simulink library "VUT_lib"  (R2023b)
settings: Solver=VariableStepAuto  StartTime=0.0  StopTime=10.0  RelTol=1e-3
undefined symbols (not defined in the file): zeroProtn
libraries: $bdroot x15
settings Model: Creator=blatak  LastModifiedBy=blatak
settings ModelReferenceCC: EnableRefExpFcnMdlSchedulingChecks=on

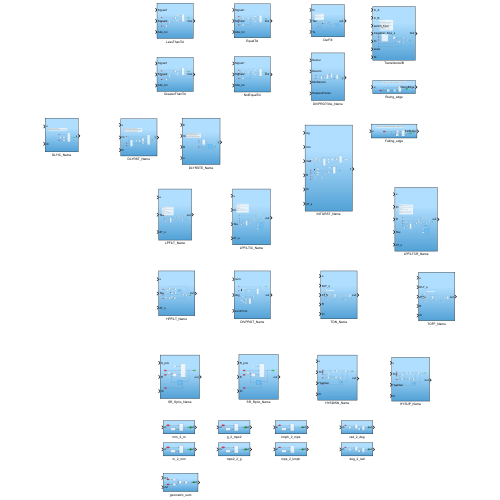
[thumbnail: Simulink's stored preview of the top-level diagram]
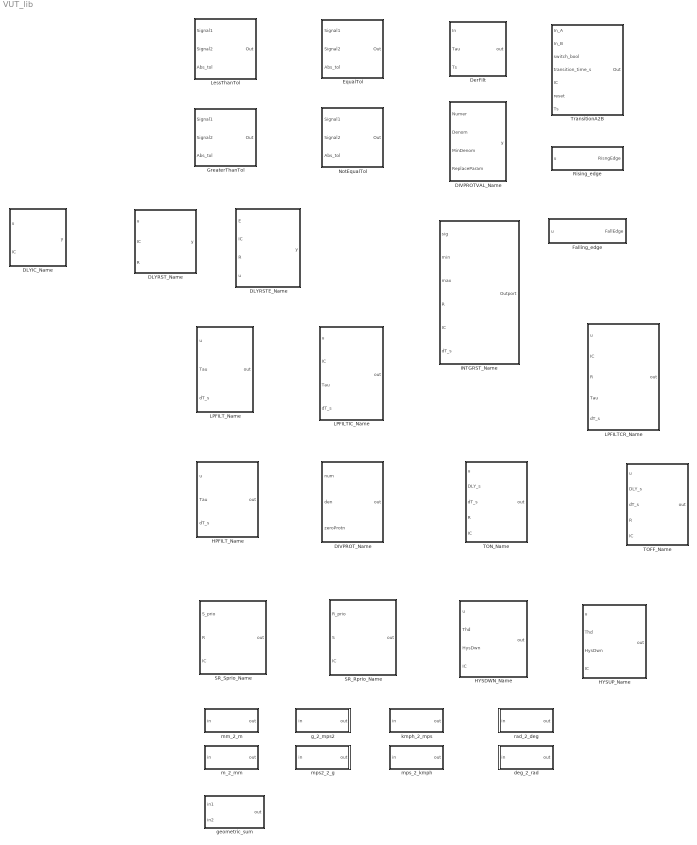
== system VUT_lib ==
  DIVPROTVAL_Name : Subsystem
  DIVPROT_Name : Subsystem
  DLYIC_Name : Subsystem
  DLYRSTE_Name : Subsystem
  DLYRST_Name : Subsystem
  DerFilt : Subsystem
  EqualTol : Subsystem
  Falling_edge : Subsystem
  GreaterThanTol : Subsystem
  HPFILT_Name : Subsystem
  HYSDWN_Name : Subsystem
  HYSUP_Name : Subsystem
  INTGRST_Name : Subsystem
  LPFILTCR_Name : Subsystem
  LPFILTIC_Name : Subsystem
  LPFILT_Name : Subsystem
  LessThanTol : Subsystem
  NotEqualTol : Subsystem
  Rising_edge : Subsystem
  SR_Rprio_Name : Subsystem
  SR_Sprio_Name : Subsystem
  TOFF_Name : Subsystem
  TON_Name : Subsystem
  TransitionA2B : Subsystem
  deg_2_rad : Subsystem
  g_2_mps2 : Subsystem
  geometric_sum : Subsystem
  kmph_2_mps : Subsystem
  m_2_mm : Subsystem
  mm_2_m : Subsystem
  mps2_2_g : Subsystem
  mps_2_kmph : Subsystem
  rad_2_deg : Subsystem

== system VUT_lib/DIVPROTVAL_Name ==
  Numer : Inport
  Denom : Inport  Port=2
  MinDenom : Inport  Port=3
  ReplaceParam : Inport  Port=4
  Abs : Abs  SaturateOnIntegerOverflow=off
  Constant : Constant  OutDataTypeStr=single
  Divide : Product  Inputs=*/  RndMeth=Zero  SaturateOnIntegerOverflow=on
  GreaterThan : RelationalOperator  Operator=>  OutDataTypeStr=boolean  RndMeth=Simplest  InputSameDT=off
  Switch : Switch  Criteria=u2 ~= 0  SaturateOnIntegerOverflow=off  InputSameDT=off
  Switch1 : Switch  Criteria=u2 ~= 0  SaturateOnIntegerOverflow=off  InputSameDT=off
  y : Outport
  wires:
  Abs/1 -> GreaterThan/1
  MinDenom/1 -> GreaterThan/2
  Constant/1 -> Switch/3
  Denom/1 -> Abs/1, Switch/1
  GreaterThan/1 -> Switch/2, Switch1/2
  Switch/1 -> Divide/2
  Numer/1 -> Divide/1
  Divide/1 -> Switch1/1
  Switch1/1 -> y/1
  ReplaceParam/1 -> Switch1/3

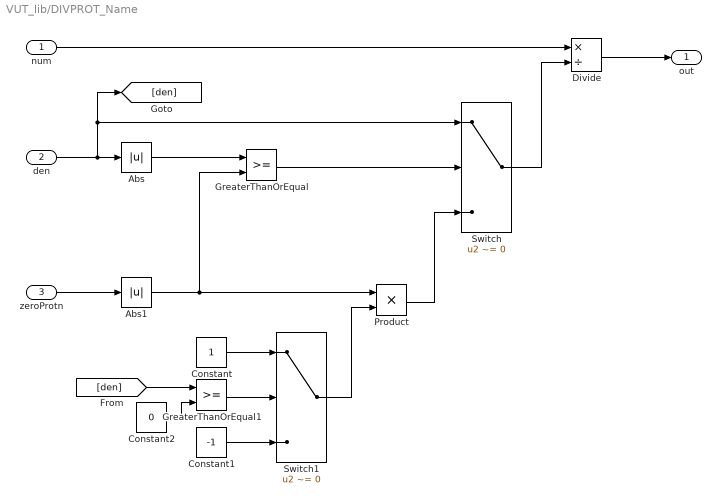
== system VUT_lib/DIVPROT_Name ==
  num : Inport
  den : Inport  Port=2
  zeroProtn : Inport  Port=3
  Abs : Abs  SaturateOnIntegerOverflow=off
  Abs1 : Abs  SaturateOnIntegerOverflow=off
  Constant : Constant  OutDataTypeStr=single
  Constant1 : Constant  Value=-1  OutDataTypeStr=single
  Constant2 : Constant  Value=0  OutDataTypeStr=single
  Divide : Product  Inputs=*/  RndMeth=Zero  SaturateOnIntegerOverflow=on
  GreaterThanOrEqual : RelationalOperator  OutDataTypeStr=boolean  RndMeth=Simplest  InputSameDT=off
  GreaterThanOrEqual1 : RelationalOperator  OutDataTypeStr=boolean  RndMeth=Simplest  InputSameDT=off
  Product : Product
  Switch : Switch  Criteria=u2 ~= 0  SaturateOnIntegerOverflow=off  InputSameDT=off
  Switch1 : Switch  Criteria=u2 ~= 0  SaturateOnIntegerOverflow=off  InputSameDT=off
  out : Outport
  wires:
  den/1 -> Switch/1, [den], Abs/1
  Abs/1 -> GreaterThanOrEqual/1
  zeroProtn/1 -> Abs1/1
  Abs1/1 -> Product/1, GreaterThanOrEqual/2
  GreaterThanOrEqual/1 -> Switch/2
  num/1 -> Divide/1
  Switch/1 -> Divide/2
  Divide/1 -> out/1
  Constant/1 -> Switch1/1
  Constant1/1 -> Switch1/3
  GreaterThanOrEqual1/1 -> Switch1/2
  [den] -> GreaterThanOrEqual1/1
  Constant2/1 -> GreaterThanOrEqual1/2
  Switch1/1 -> Product/2
  Product/1 -> Switch/3

== system VUT_lib/DLYIC_Name ==
  note: Unit delay External Initial Condition
      | Normally, the output is the signal delayed by one sample period.
      | Initial condition is given by the signal IC.
  u : Inport
  IC : Inport  Port=2
  Constant : Constant  Value=false  OutDataTypeStr=boolean
  Switch : Switch  Criteria=u2 ~= 0  SaturateOnIntegerOverflow=off  InputSameDT=off
  Unit Delay : UnitDelay  SampleTime=-1  HasFrameUpgradeWarning=on
  Unit Delay1 : UnitDelay  InitialCondition=true  SampleTime=-1  HasFrameUpgradeWarning=on
  y : Outport
  wires:
  u/1 -> Unit Delay/1
  Unit Delay/1 -> Switch/3
  IC/1 -> Switch/1
  Constant/1 -> Unit Delay1/1
  Unit Delay1/1 -> Switch/2
  Switch/1 -> y/1

== system VUT_lib/DLYRSTE_Name ==
  note: Unit Delay Resettable External Initial Condition
      | Normally, the output is the signal delayed by one sample period.
      | When the reset signal R is true, the state and the output are always set equal to the initial condition signal IC. This reset action is vectorized and supports scalar expansion.
      | When the enable signal is false, the block is disabled, and the state and the output values do not change except for resets. The enable action is vectoriyed and supports scalar expansion.
  E : Inport
  IC : Inport  Port=2
  R : Inport  Port=3
  u : Inport  Port=4
  DLYRST_Name : $bdroot/DLYRST_Name  SystemSampleTime=-1  VariantActivationTime=update diagram  Latency=0  AutoFrameSizeCalculation=off
  Switch : Switch  Criteria=u2 ~= 0  SaturateOnIntegerOverflow=off  InputSameDT=off
  y : Outport
  wires:
  E/1 -> Switch/2
  Switch/1 -> DLYRST_Name/1
  IC/1 -> DLYRST_Name/2
  R/1 -> DLYRST_Name/3
  DLYRST_Name/1 -> Switch/3, y/1
  u/1 -> Switch/1

== system VUT_lib/DLYRST_Name ==
  note: Unit Delay Resettable External Initial Condition
      | Normally, the output is the signal delayed by one sample period.
      | When the reset signal R is true, the state and the output are always set equal to the initial condition signal IC. This reset action is vectorized and supports scalar expansion.
  u : Inport
  IC : Inport  Port=2
  R : Inport  Port=3
  Constant : Constant  Value=false  OutDataTypeStr=boolean
  Logical Operator : Logic  Operator=OR  AllPortsSameDT=off  OutDataTypeStr=boolean
  Switch : Switch  Criteria=u2 ~= 0  SaturateOnIntegerOverflow=off  InputSameDT=off
  Switch1 : Switch  Criteria=u2 ~= 0  SaturateOnIntegerOverflow=off  InputSameDT=off
  Unit Delay : UnitDelay  InitialCondition=true  SampleTime=-1  HasFrameUpgradeWarning=on
  Unit Delay1 : UnitDelay  SampleTime=-1  HasFrameUpgradeWarning=on
  y : Outport
  wires:
  u/1 -> Switch/3
  R/1 -> Logical Operator/1, Switch/2
  Constant/1 -> Unit Delay/1
  Unit Delay/1 -> Logical Operator/2
  Switch/1 -> Unit Delay1/1
  Unit Delay1/1 -> Switch1/3
  Logical Operator/1 -> Switch1/2
  IC/1 -> Switch/1, Switch1/1
  Switch1/1 -> y/1

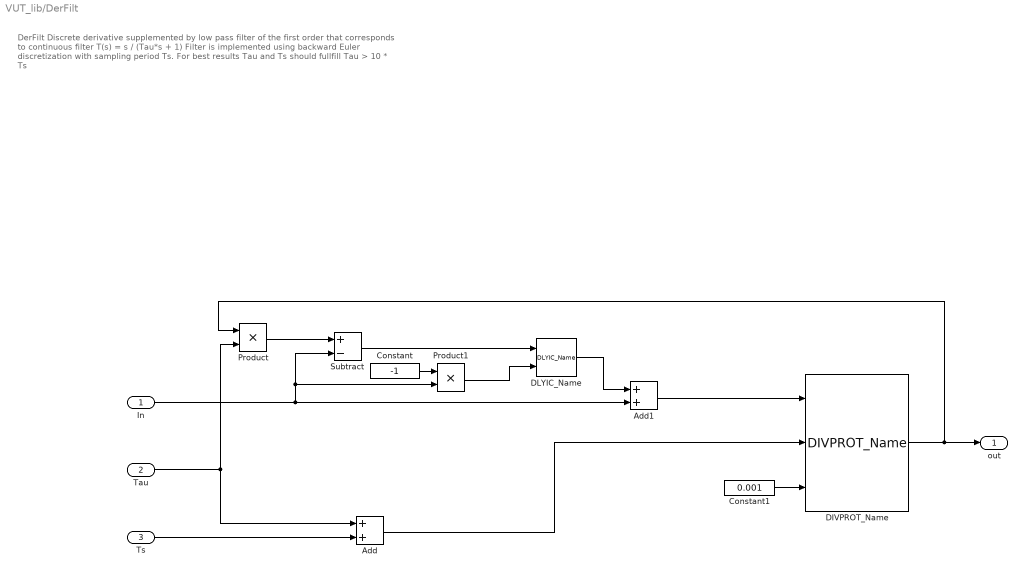
== system VUT_lib/DerFilt ==
  note: DerFilt
      |
      | Discrete derivative supplemented by low pass filter of the first
      | order that corresponds to continuous filter
      |
      | T(s) = s / (Tau*s + 1)
      |
      | Filter is implemented using backward Euler discretization with
      | sampling period Ts.
      |
      | For best results Tau and Ts should fullfill
      |
      | Tau > 10 * Ts
  In : Inport
  Tau : Inport  Port=2
  Ts : Inport  Port=3
  Add : Sum
  Add1 : Sum
  Constant : Constant  Value=-1  OutDataTypeStr=single
  Constant1 : Constant  Value=0.001  OutDataTypeStr=single
  DIVPROT_Name : $bdroot/DIVPROT_Name  SystemSampleTime=-1  VariantActivationTime=update diagram  Latency=0  AutoFrameSizeCalculation=off
  DLYIC_Name : $bdroot/DLYIC_Name  SystemSampleTime=-1  VariantActivationTime=update diagram  Latency=0  AutoFrameSizeCalculation=off
  Product : Product
  Product1 : Product
  Subtract : Sum  Inputs=+-
  out : Outport
  wires:
  Ts/1 -> Add/2
  Tau/1 -> Product/2, Add/1
  Product/1 -> Subtract/1
  In/1 -> Product1/2, Subtract/2, Add1/2
  Product1/1 -> DLYIC_Name/2
  Subtract/1 -> DLYIC_Name/1
  Constant/1 -> Product1/1
  Add1/1 -> DIVPROT_Name/1
  Add/1 -> DIVPROT_Name/2
  DIVPROT_Name/1 -> Product/1, out/1
  DLYIC_Name/1 -> Add1/1
  Constant1/1 -> DIVPROT_Name/3

== system VUT_lib/EqualTol ==
  Signal1 : Inport
  Signal2 : Inport  Port=2
  Abs_tol : Inport  Port=3
  Abs : Abs  SaturateOnIntegerOverflow=off
  Abs1 : Abs  SaturateOnIntegerOverflow=off
  Add : Sum  Inputs=+-
  Constant : Constant  Value=true  OutDataTypeStr=boolean
  Constant1 : Constant  Value=false  OutDataTypeStr=boolean
  LessThanOrEqual : RelationalOperator  Operator=<=  OutDataTypeStr=boolean  RndMeth=Simplest  InputSameDT=off
  Switch : Switch  Criteria=u2 ~= 0  SaturateOnIntegerOverflow=off  InputSameDT=off
  Out : Outport
  wires:
  Abs_tol/1 -> Abs/1
  Signal1/1 -> Add/1
  Signal2/1 -> Add/2
  Add/1 -> Abs1/1
  Abs1/1 -> LessThanOrEqual/1
  Abs/1 -> LessThanOrEqual/2
  LessThanOrEqual/1 -> Switch/2
  Constant/1 -> Switch/1
  Constant1/1 -> Switch/3
  Switch/1 -> Out/1

== system VUT_lib/Falling_edge ==
  note: This block is used to detect falling edge on logical signal
  u : Inport
  Logical Operator : Logic  Operator=NOT  AllPortsSameDT=off  OutDataTypeStr=boolean
  Logical Operator1 : Logic  AllPortsSameDT=off  OutDataTypeStr=boolean
  Unit Delay : UnitDelay  SampleTime=-1  HasFrameUpgradeWarning=on
  FallEdge : Outport
  wires:
  u/1 -> Unit Delay/1, Logical Operator/1
  Logical Operator1/1 -> FallEdge/1
  Unit Delay/1 -> Logical Operator1/2
  Logical Operator/1 -> Logical Operator1/1

== system VUT_lib/GreaterThanTol ==
  Signal1 : Inport
  Signal2 : Inport  Port=2
  Abs_tol : Inport  Port=3
  Abs : Abs  SaturateOnIntegerOverflow=off
  Add : Sum
  Constant : Constant  Value=true  OutDataTypeStr=boolean
  Constant1 : Constant  Value=false  OutDataTypeStr=boolean
  GreaterThan : RelationalOperator  Operator=>  OutDataTypeStr=boolean  RndMeth=Simplest  InputSameDT=off
  Switch : Switch  Criteria=u2 ~= 0  SaturateOnIntegerOverflow=off  InputSameDT=off
  Out : Outport
  wires:
  Abs_tol/1 -> Abs/1
  Abs/1 -> Add/2
  Constant/1 -> Switch/1
  Add/1 -> GreaterThan/2
  Switch/1 -> Out/1
  Signal1/1 -> GreaterThan/1
  Signal2/1 -> Add/1
  Constant1/1 -> Switch/3
  GreaterThan/1 -> Switch/2

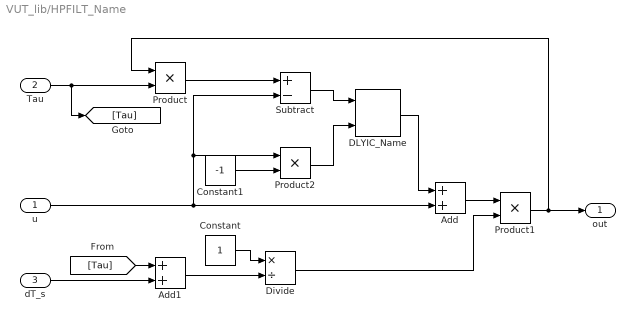
== system VUT_lib/HPFILT_Name ==
  u : Inport
  Tau : Inport  Port=2
  dT_s : Inport  Port=3
  Add : Sum
  Add1 : Sum
  Constant : Constant  OutDataTypeStr=single
  Constant1 : Constant  Value=-1  OutDataTypeStr=single
  DLYIC_Name : $bdroot/DLYIC_Name  SystemSampleTime=-1  VariantActivationTime=update diagram  Latency=0  AutoFrameSizeCalculation=off
  Divide : Product  Inputs=*/  RndMeth=Zero  SaturateOnIntegerOverflow=on
  Product : Product
  Product1 : Product
  Product2 : Product
  Subtract : Sum  Inputs=+-
  out : Outport
  wires:
  Tau/1 -> [Tau], Product/2
  Product/1 -> Subtract/1
  u/1 -> Product2/1, Subtract/2, Add/2
  Add/1 -> Product1/1
  dT_s/1 -> Add1/2
  [Tau] -> Add1/1
  Add1/1 -> Divide/2
  Constant/1 -> Divide/1
  Divide/1 -> Product1/2
  Product1/1 -> Product/1, out/1
  Constant1/1 -> Product2/2
  Subtract/1 -> DLYIC_Name/1
  Product2/1 -> DLYIC_Name/2
  DLYIC_Name/1 -> Add/1

== system VUT_lib/HYSDWN_Name ==
  u : Inport
  Thd : Inport  Port=2
  HysDwn : Inport  Port=3
  IC : Inport  Port=4
  DLYIC_Name : $bdroot/DLYIC_Name  SystemSampleTime=-1  VariantActivationTime=update diagram  Latency=0  AutoFrameSizeCalculation=off
  GreaterThanOrEqual : RelationalOperator  OutDataTypeStr=boolean  RndMeth=Simplest  InputSameDT=off
  GreaterThanOrEqual1 : RelationalOperator  OutDataTypeStr=boolean  RndMeth=Simplest  InputSameDT=off
  Logical Operator : Logic  AllPortsSameDT=off  OutDataTypeStr=boolean
  Logical Operator1 : Logic  Operator=OR  AllPortsSameDT=off  OutDataTypeStr=boolean
  Subtract : Sum  Inputs=+-
  out : Outport
  wires:
  u/1 -> GreaterThanOrEqual1/1, GreaterThanOrEqual/1
  HysDwn/1 -> Subtract/2
  Thd/1 -> [Thd], Subtract/1
  Subtract/1 -> GreaterThanOrEqual/2
  [Thd] -> GreaterThanOrEqual1/2
  GreaterThanOrEqual/1 -> Logical Operator/1
  DLYIC_Name/1 -> Logical Operator/2
  IC/1 -> DLYIC_Name/2
  GreaterThanOrEqual1/1 -> Logical Operator1/1
  Logical Operator/1 -> Logical Operator1/2
  Logical Operator1/1 -> DLYIC_Name/1, out/1

== system VUT_lib/HYSUP_Name ==
  u : Inport
  Thd : Inport  Port=2
  HysDwn : Inport  Port=3
  IC : Inport  Port=4
  DLYIC_Name : $bdroot/DLYIC_Name  SystemSampleTime=-1  VariantActivationTime=update diagram  Latency=0  AutoFrameSizeCalculation=off
  GreaterThanOrEqual : RelationalOperator  Operator=<=  OutDataTypeStr=boolean  RndMeth=Simplest  InputSameDT=off
  GreaterThanOrEqual1 : RelationalOperator  Operator=<=  OutDataTypeStr=boolean  RndMeth=Simplest  InputSameDT=off
  Logical Operator : Logic  AllPortsSameDT=off  OutDataTypeStr=boolean
  Logical Operator1 : Logic  Operator=OR  AllPortsSameDT=off  OutDataTypeStr=boolean
  Subtract : Sum  Inputs=+-
  out : Outport
  wires:
  Thd/1 -> [Thd], Subtract/1
  GreaterThanOrEqual1/1 -> Logical Operator1/1
  Logical Operator/1 -> Logical Operator1/2
  IC/1 -> DLYIC_Name/2
  u/1 -> GreaterThanOrEqual1/1, GreaterThanOrEqual/1
  HysDwn/1 -> Subtract/2
  GreaterThanOrEqual/1 -> Logical Operator/1
  Logical Operator1/1 -> DLYIC_Name/1, out/1
  Subtract/1 -> GreaterThanOrEqual/2
  DLYIC_Name/1 -> Logical Operator/2
  [Thd] -> GreaterThanOrEqual1/2

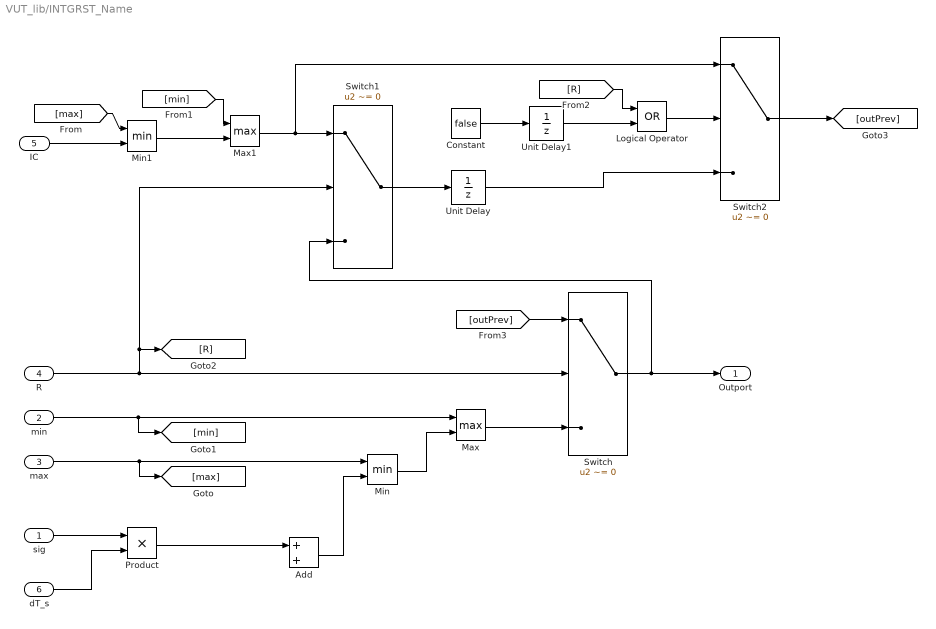
== system VUT_lib/INTGRST_Name ==
  sig : Inport
  min : Inport  Port=2
  max : Inport  Port=3
  R : Inport  Port=4
  IC : Inport  Port=5
  dT_s : Inport  Port=6
  Add : Sum
  Constant : Constant  Value=false  OutDataTypeStr=boolean
  Logical Operator : Logic  Operator=OR  AllPortsSameDT=off  OutDataTypeStr=boolean
  Max : MinMax  Function=max  Inputs=2
  Max1 : MinMax  Function=max  Inputs=2
  Min : MinMax  Inputs=2
  Min1 : MinMax  Inputs=2
  Product : Product
  Switch : Switch  Criteria=u2 ~= 0  SaturateOnIntegerOverflow=off  InputSameDT=off
  Switch1 : Switch  Criteria=u2 ~= 0  SaturateOnIntegerOverflow=off  InputSameDT=off
  Switch2 : Switch  Criteria=u2 ~= 0  SaturateOnIntegerOverflow=off  InputSameDT=off
  Unit Delay : UnitDelay  SampleTime=-1  HasFrameUpgradeWarning=on
  Unit Delay1 : UnitDelay  InitialCondition=true  SampleTime=-1  HasFrameUpgradeWarning=on
  Outport : Outport
  wires:
  sig/1 -> Product/1
  dT_s/1 -> Product/2
  Product/1 -> Add/1
  max/1 -> [max], Min/1
  Add/1 -> Min/2
  Min/1 -> Max/2
  min/1 -> [min], Max/1
  Max/1 -> Switch/3
  R/1 -> Switch1/2, [R], Switch/2
  IC/1 -> Min1/2
  [max] -> Min1/1
  Min1/1 -> Max1/2
  [min] -> Max1/1
  Max1/1 -> Switch2/1, Switch1/1
  Switch/1 -> Switch1/3, Outport/1
  Switch1/1 -> Unit Delay/1
  Constant/1 -> Unit Delay1/1
  Unit Delay1/1 -> Logical Operator/2
  [R] -> Logical Operator/1
  Logical Operator/1 -> Switch2/2
  Unit Delay/1 -> Switch2/3
  Switch2/1 -> [outPrev]
  [outPrev] -> Switch/1

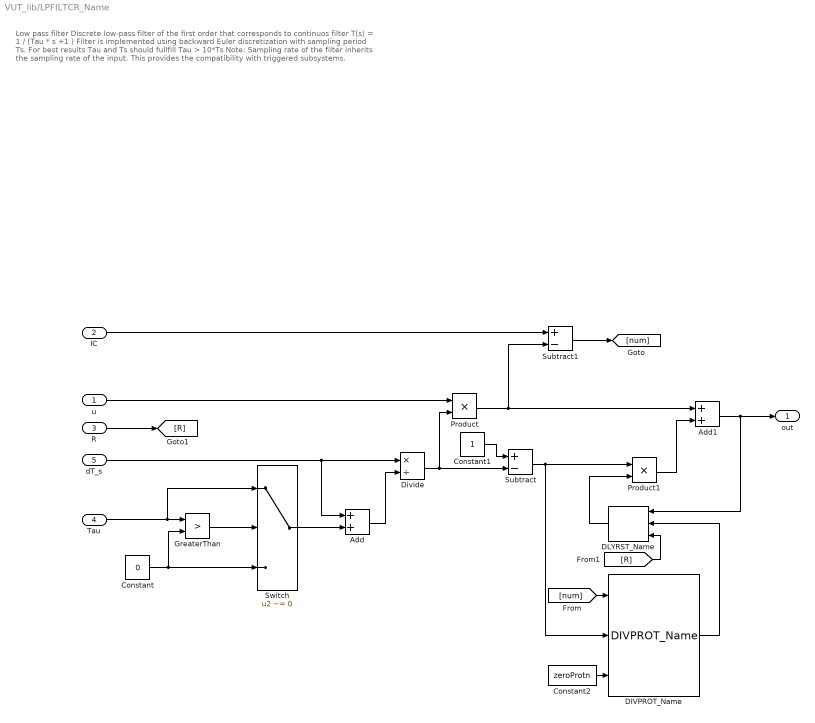
== system VUT_lib/LPFILTCR_Name ==
  note: Low pass filter
      | Discrete low-pass filter of the first order that corresponds to
      | continuos filter
      |
      | T(s) = 1 / (Tau * s +1 )
      |
      | Filter is implemented using backward Euler discretization with sampling period Ts.
      |
      | For best results Tau and Ts should fullfill
      | Tau > 10*Ts
      |
      | Note: Sampling rate of the filter inherits the sampling rate of the input. This provides the compatibility with triggered subsystems.
  u : Inport
  IC : Inport  Port=2
  R : Inport  Port=3
  Tau : Inport  Port=4
  dT_s : Inport  Port=5
  Add : Sum
  Add1 : Sum
  Constant : Constant  Value=0
  Constant1 : Constant  OutDataTypeStr=single
  Constant2 : Constant  Value=zeroProtn
  DIVPROT_Name : $bdroot/DIVPROT_Name  SystemSampleTime=-1  VariantActivationTime=update diagram  Latency=0  AutoFrameSizeCalculation=off
  DLYRST_Name : $bdroot/DLYRST_Name  SystemSampleTime=-1  VariantActivationTime=update diagram  Latency=0  AutoFrameSizeCalculation=off
  Divide : Product  Inputs=*/  RndMeth=Zero  SaturateOnIntegerOverflow=on
  GreaterThan : RelationalOperator  Operator=>  OutDataTypeStr=boolean  RndMeth=Simplest  InputSameDT=off
  Product : Product
  Product1 : Product
  Subtract : Sum  Inputs=+-
  Subtract1 : Sum  Inputs=+-
  Switch : Switch  Criteria=u2 ~= 0  SaturateOnIntegerOverflow=off  InputSameDT=off
  out : Outport
  wires:
  Divide/1 -> Subtract/2, Product/2
  u/1 -> Product/1
  dT_s/1 -> Add/1, Divide/1
  Subtract/1 -> DIVPROT_Name/2, Product1/1
  DIVPROT_Name/1 -> DLYRST_Name/2
  GreaterThan/1 -> Switch/2
  Add1/1 -> DLYRST_Name/1, out/1
  Constant1/1 -> Subtract/1
  Switch/1 -> Add/2
  Add/1 -> Divide/2
  Product1/1 -> Add1/2
  [num] -> DIVPROT_Name/1
  DLYRST_Name/1 -> Product1/2
  Tau/1 -> Switch/1, GreaterThan/1
  Constant2/1 -> DIVPROT_Name/3
  Subtract1/1 -> [num]
  Constant/1 -> Switch/3, GreaterThan/2
  IC/1 -> Subtract1/1
  Product/1 -> Subtract1/2, Add1/1
  R/1 -> [R]
  [R] -> DLYRST_Name/3

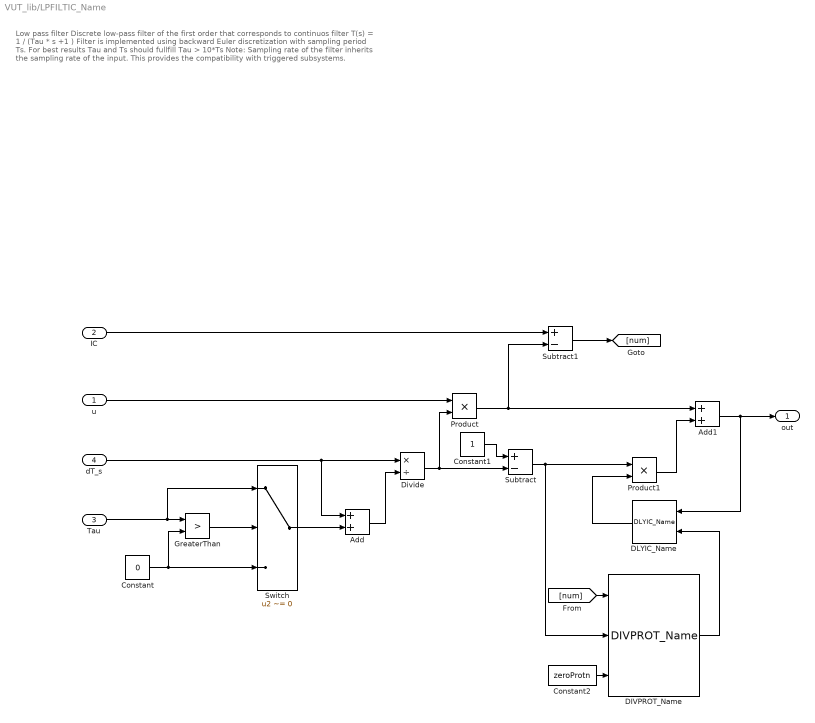
== system VUT_lib/LPFILTIC_Name ==
  note: Low pass filter
      | Discrete low-pass filter of the first order that corresponds to
      | continuos filter
      |
      | T(s) = 1 / (Tau * s +1 )
      |
      | Filter is implemented using backward Euler discretization with sampling period Ts.
      |
      | For best results Tau and Ts should fullfill
      | Tau > 10*Ts
      |
      | Note: Sampling rate of the filter inherits the sampling rate of the input. This provides the compatibility with triggered subsystems.
  u : Inport
  IC : Inport  Port=2
  Tau : Inport  Port=3
  dT_s : Inport  Port=4
  Add : Sum
  Add1 : Sum
  Constant : Constant  Value=0
  Constant1 : Constant  OutDataTypeStr=single
  Constant2 : Constant  Value=zeroProtn
  DIVPROT_Name : $bdroot/DIVPROT_Name  SystemSampleTime=-1  VariantActivationTime=update diagram  Latency=0  AutoFrameSizeCalculation=off
  DLYIC_Name : $bdroot/DLYIC_Name  SystemSampleTime=-1  VariantActivationTime=update diagram  Latency=0  AutoFrameSizeCalculation=off
  Divide : Product  Inputs=*/  RndMeth=Zero  SaturateOnIntegerOverflow=on
  GreaterThan : RelationalOperator  Operator=>  OutDataTypeStr=boolean  RndMeth=Simplest  InputSameDT=off
  Product : Product
  Product1 : Product
  Subtract : Sum  Inputs=+-
  Subtract1 : Sum  Inputs=+-
  Switch : Switch  Criteria=u2 ~= 0  SaturateOnIntegerOverflow=off  InputSameDT=off
  out : Outport
  wires:
  Product1/1 -> Add1/2
  Product/1 -> Subtract1/2, Add1/1
  Switch/1 -> Add/2
  Add1/1 -> DLYIC_Name/1, out/1
  Tau/1 -> Switch/1, GreaterThan/1
  Add/1 -> Divide/2
  GreaterThan/1 -> Switch/2
  dT_s/1 -> Add/1, Divide/1
  Subtract/1 -> DIVPROT_Name/2, Product1/1
  Constant/1 -> Switch/3, GreaterThan/2
  u/1 -> Product/1
  Constant1/1 -> Subtract/1
  DLYIC_Name/1 -> Product1/2
  Divide/1 -> Subtract/2, Product/2
  DIVPROT_Name/1 -> DLYIC_Name/2
  IC/1 -> Subtract1/1
  Subtract1/1 -> [num]
  [num] -> DIVPROT_Name/1
  Constant2/1 -> DIVPROT_Name/3

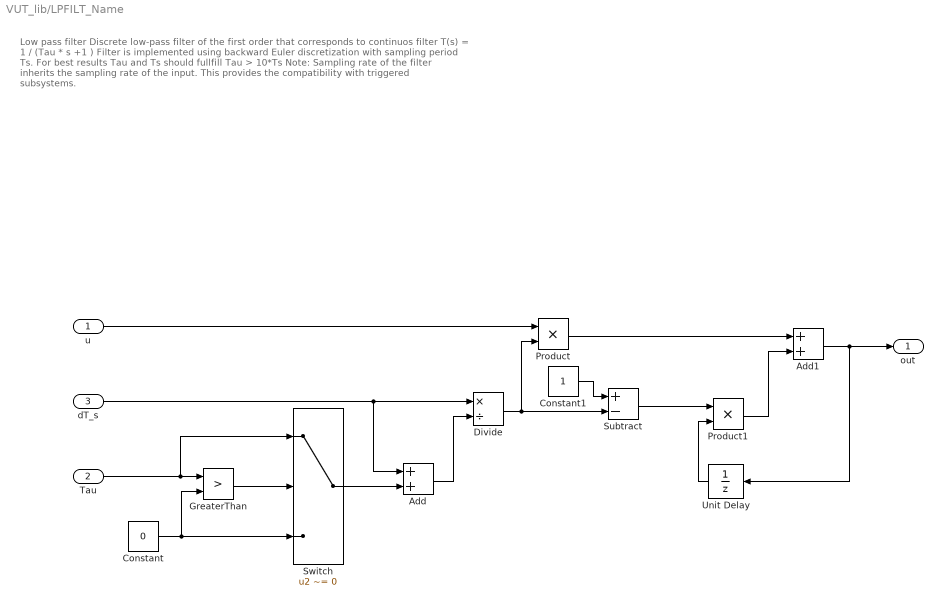
== system VUT_lib/LPFILT_Name ==
  note: Low pass filter
      | Discrete low-pass filter of the first order that corresponds to
      | continuos filter
      |
      | T(s) = 1 / (Tau * s +1 )
      |
      | Filter is implemented using backward Euler discretization with sampling period Ts.
      |
      | For best results Tau and Ts should fullfill
      | Tau > 10*Ts
      |
      | Note: Sampling rate of the filter inherits the sampling rate of the input. This provides the compatibility with triggered subsystems.
  u : Inport
  Tau : Inport  Port=2
  dT_s : Inport  Port=3
  Add : Sum
  Add1 : Sum
  Constant : Constant  Value=0
  Constant1 : Constant  OutDataTypeStr=single
  Divide : Product  Inputs=*/  RndMeth=Zero  SaturateOnIntegerOverflow=on
  GreaterThan : RelationalOperator  Operator=>  OutDataTypeStr=boolean  RndMeth=Simplest  InputSameDT=off
  Product : Product
  Product1 : Product
  Subtract : Sum  Inputs=+-
  Switch : Switch  Criteria=u2 ~= 0  SaturateOnIntegerOverflow=off  InputSameDT=off
  Unit Delay : UnitDelay  SampleTime=-1  HasFrameUpgradeWarning=on
  out : Outport
  wires:
  Tau/1 -> Switch/1, GreaterThan/1
  Constant/1 -> Switch/3, GreaterThan/2
  GreaterThan/1 -> Switch/2
  Switch/1 -> Add/2
  dT_s/1 -> Add/1, Divide/1
  Add/1 -> Divide/2
  Divide/1 -> Subtract/2, Product/2
  u/1 -> Product/1
  Constant1/1 -> Subtract/1
  Subtract/1 -> Product1/1
  Unit Delay/1 -> Product1/2
  Product/1 -> Add1/1
  Product1/1 -> Add1/2
  Add1/1 -> Unit Delay/1, out/1

== system VUT_lib/LessThanTol ==
  Signal1 : Inport
  Signal2 : Inport  Port=2
  Abs_tol : Inport  Port=3
  Abs : Abs  SaturateOnIntegerOverflow=off
  Add : Sum
  Constant : Constant  Value=true  OutDataTypeStr=boolean
  Constant1 : Constant  Value=false  OutDataTypeStr=boolean
  Less Than : RelationalOperator  Operator=<  OutDataTypeStr=boolean  RndMeth=Simplest  InputSameDT=off
  Switch : Switch  Criteria=u2 ~= 0  SaturateOnIntegerOverflow=off  InputSameDT=off
  Out : Outport
  wires:
  Signal1/1 -> Less Than/1
  Signal2/1 -> Add/1
  Abs_tol/1 -> Abs/1
  Abs/1 -> Add/2
  Add/1 -> Less Than/2
  Less Than/1 -> Switch/2
  Switch/1 -> Out/1
  Constant/1 -> Switch/1
  Constant1/1 -> Switch/3

== system VUT_lib/NotEqualTol ==
  Signal1 : Inport
  Signal2 : Inport  Port=2
  Abs_tol : Inport  Port=3
  Abs : Abs  SaturateOnIntegerOverflow=off
  Abs1 : Abs  SaturateOnIntegerOverflow=off
  Add : Sum  Inputs=+-
  Constant : Constant  Value=true  OutDataTypeStr=boolean
  Constant1 : Constant  Value=false  OutDataTypeStr=boolean
  LessThanOrEqual : RelationalOperator  Operator=>  OutDataTypeStr=boolean  RndMeth=Simplest  InputSameDT=off
  Switch : Switch  Criteria=u2 ~= 0  SaturateOnIntegerOverflow=off  InputSameDT=off
  Out : Outport
  wires:
  Abs_tol/1 -> Abs/1
  Signal2/1 -> Add/2
  LessThanOrEqual/1 -> Switch/2
  Switch/1 -> Out/1
  Constant1/1 -> Switch/3
  Constant/1 -> Switch/1
  Signal1/1 -> Add/1
  Abs/1 -> LessThanOrEqual/2
  Add/1 -> Abs1/1
  Abs1/1 -> LessThanOrEqual/1

== system VUT_lib/Rising_edge ==
  note: This block is used to detect rising edge on logical signal
  u : Inport
  Logical Operator : Logic  Operator=NOT  AllPortsSameDT=off  OutDataTypeStr=boolean
  Logical Operator1 : Logic  AllPortsSameDT=off  OutDataTypeStr=boolean
  Unit Delay : UnitDelay  SampleTime=-1  HasFrameUpgradeWarning=on
  RisngEdge : Outport
  wires:
  Unit Delay/1 -> Logical Operator/1
  Logical Operator/1 -> Logical Operator1/2
  u/1 -> Logical Operator1/1, Unit Delay/1
  Logical Operator1/1 -> RisngEdge/1

== system VUT_lib/SR_Rprio_Name ==
  R_prio : Inport
  S : Inport  Port=2
  IC : Inport  Port=3
  Constant : Constant  Value=false  OutDataTypeStr=boolean
  Constant1 : Constant  Value=true  OutDataTypeStr=boolean
  DLYIC_Name : $bdroot/DLYIC_Name  SystemSampleTime=-1  VariantActivationTime=update diagram  Latency=0  AutoFrameSizeCalculation=off
  Switch : Switch  Criteria=u2 ~= 0  SaturateOnIntegerOverflow=off  InputSameDT=off
  Switch1 : Switch  Criteria=u2 ~= 0  SaturateOnIntegerOverflow=off  InputSameDT=off
  out : Outport
  wires:
  Switch1/1 -> Switch/3
  R_prio/1 -> Switch/2
  Constant/1 -> Switch/1
  IC/1 -> DLYIC_Name/2
  Constant1/1 -> Switch1/1
  DLYIC_Name/1 -> Switch1/3
  S/1 -> Switch1/2
  Switch/1 -> DLYIC_Name/1, out/1

== system VUT_lib/SR_Sprio_Name ==
  S_prio : Inport
  R : Inport  Port=2
  IC : Inport  Port=3
  Constant : Constant  Value=true  OutDataTypeStr=boolean
  Constant1 : Constant  Value=false  OutDataTypeStr=boolean
  DLYIC_Name : $bdroot/DLYIC_Name  SystemSampleTime=-1  VariantActivationTime=update diagram  Latency=0  AutoFrameSizeCalculation=off
  Switch : Switch  Criteria=u2 ~= 0  SaturateOnIntegerOverflow=off  InputSameDT=off
  Switch1 : Switch  Criteria=u2 ~= 0  SaturateOnIntegerOverflow=off  InputSameDT=off
  out : Outport
  wires:
  S_prio/1 -> Switch/2
  Switch/1 -> DLYIC_Name/1, out/1
  Constant/1 -> Switch/1
  Switch1/1 -> Switch/3
  R/1 -> Switch1/2
  Constant1/1 -> Switch1/1
  IC/1 -> DLYIC_Name/2
  DLYIC_Name/1 -> Switch1/3

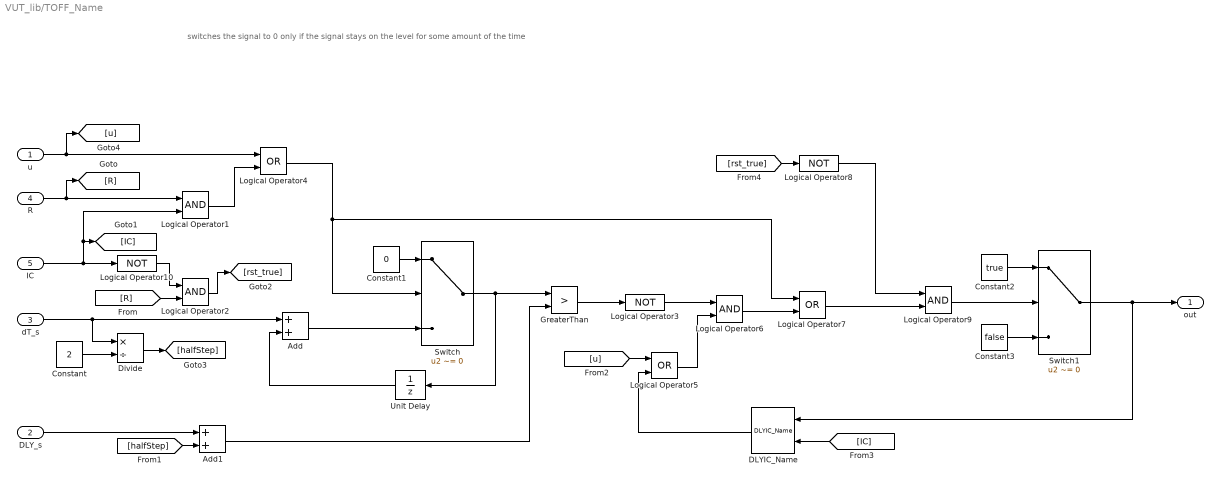
== system VUT_lib/TOFF_Name ==
  note: switches the signal to 0 only if the signal stays on the level for some amount of the time
  u : Inport
  DLY_s : Inport  Port=2
  dT_s : Inport  Port=3
  R : Inport  Port=4
  IC : Inport  Port=5
  Add : Sum
  Add1 : Sum
  Constant : Constant  Value=2  OutDataTypeStr=single
  Constant1 : Constant  Value=0  OutDataTypeStr=single
  Constant2 : Constant  Value=true  OutDataTypeStr=boolean
  Constant3 : Constant  Value=false  OutDataTypeStr=boolean
  DLYIC_Name : $bdroot/DLYIC_Name  SystemSampleTime=-1  VariantActivationTime=update diagram  Latency=0  AutoFrameSizeCalculation=off
  Divide : Product  Inputs=*/  RndMeth=Zero  SaturateOnIntegerOverflow=on
  GreaterThan : RelationalOperator  Operator=>  OutDataTypeStr=boolean  RndMeth=Simplest  InputSameDT=off
  Logical Operator{1..2,6,9} (4 alike) : Logic  AllPortsSameDT=off  OutDataTypeStr=boolean
  Logical Operator10 : Logic  Operator=NOT  AllPortsSameDT=off  OutDataTypeStr=boolean
  Logical Operator3 : Logic  Operator=NOT  AllPortsSameDT=off  OutDataTypeStr=boolean
  Logical Operator4 : Logic  Operator=OR  AllPortsSameDT=off  OutDataTypeStr=boolean
  Logical Operator5 : Logic  Operator=OR  AllPortsSameDT=off  OutDataTypeStr=boolean
  Logical Operator7 : Logic  Operator=OR  AllPortsSameDT=off  OutDataTypeStr=boolean
  Logical Operator8 : Logic  Operator=NOT  AllPortsSameDT=off  OutDataTypeStr=boolean
  Switch : Switch  Criteria=u2 ~= 0  SaturateOnIntegerOverflow=off  InputSameDT=off
  Switch1 : Switch  Criteria=u2 ~= 0  SaturateOnIntegerOverflow=off  InputSameDT=off
  Unit Delay : UnitDelay  SampleTime=-1  HasFrameUpgradeWarning=on
  out : Outport
  wires:
  IC/1 -> Logical Operator1/2, [IC], Logical Operator10/1
  Switch/1 -> Unit Delay/1, GreaterThan/1
  [rst_true] -> Logical Operator8/1
  Logical Operator9/1 -> Switch1/2
  Logical Operator5/1 -> Logical Operator6/2
  Divide/1 -> [halfStep]
  DLYIC_Name/1 -> Logical Operator5/2
  dT_s/1 -> Divide/1, Add/1
  Unit Delay/1 -> Add/2
  [R] -> Logical Operator2/2
  R/1 -> [R], Logical Operator1/1
  Constant/1 -> Divide/2
  Constant1/1 -> Switch/1
  Logical Operator6/1 -> Logical Operator7/2
  Add1/1 -> GreaterThan/2
  Logical Operator2/1 -> [rst_true]
  Logical Operator4/1 -> Logical Operator7/1, Switch/2
  Add/1 -> Switch/3
  DLY_s/1 -> Add1/1
  Logical Operator7/1 -> Logical Operator9/2
  [halfStep] -> Add1/2
  Constant3/1 -> Switch1/3
  Logical Operator1/1 -> Logical Operator4/2
  Constant2/1 -> Switch1/1
  [IC] -> DLYIC_Name/2
  GreaterThan/1 -> Logical Operator3/1
  [u] -> Logical Operator5/1
  u/1 -> Logical Operator4/1, [u]
  Switch1/1 -> DLYIC_Name/1, out/1
  Logical Operator10/1 -> Logical Operator2/1
  Logical Operator3/1 -> Logical Operator6/1
  Logical Operator8/1 -> Logical Operator9/1

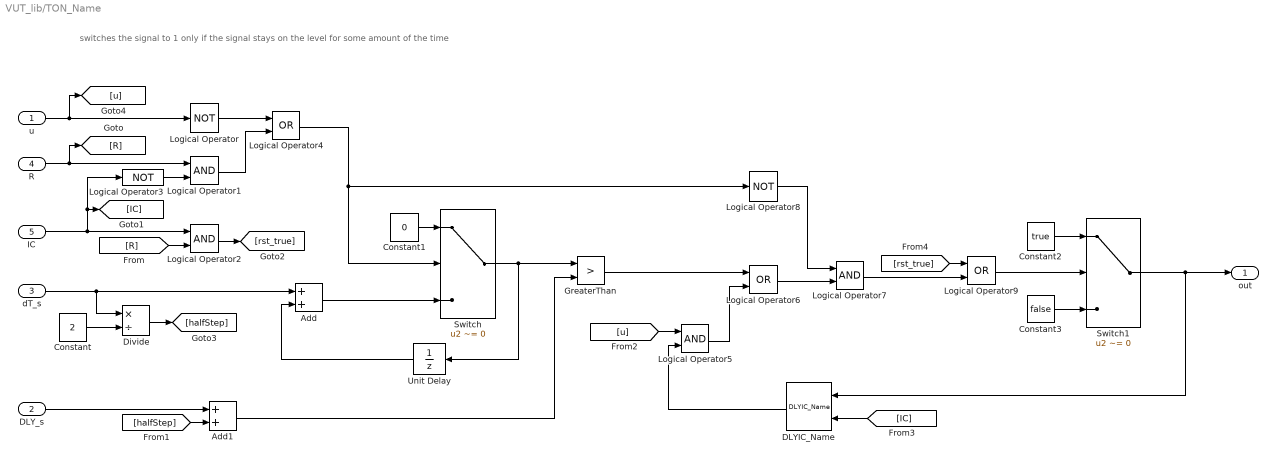
== system VUT_lib/TON_Name ==
  note: switches the signal to 1 only if the signal stays on the level for some amount of the time
  u : Inport
  DLY_s : Inport  Port=2
  dT_s : Inport  Port=3
  R : Inport  Port=4
  IC : Inport  Port=5
  Add : Sum
  Add1 : Sum
  Constant : Constant  Value=2  OutDataTypeStr=single
  Constant1 : Constant  Value=0  OutDataTypeStr=single
  Constant2 : Constant  Value=true  OutDataTypeStr=boolean
  Constant3 : Constant  Value=false  OutDataTypeStr=boolean
  DLYIC_Name : $bdroot/DLYIC_Name  SystemSampleTime=-1  VariantActivationTime=update diagram  Latency=0  AutoFrameSizeCalculation=off
  Divide : Product  Inputs=*/  RndMeth=Zero  SaturateOnIntegerOverflow=on
  GreaterThan : RelationalOperator  Operator=>  OutDataTypeStr=boolean  RndMeth=Simplest  InputSameDT=off
  Logical Operator : Logic  Operator=NOT  AllPortsSameDT=off  OutDataTypeStr=boolean
  Logical Operator{1..2,5,7} (4 alike) : Logic  AllPortsSameDT=off  OutDataTypeStr=boolean
  Logical Operator3 : Logic  Operator=NOT  AllPortsSameDT=off  OutDataTypeStr=boolean
  Logical Operator4 : Logic  Operator=OR  AllPortsSameDT=off  OutDataTypeStr=boolean
  Logical Operator6 : Logic  Operator=OR  AllPortsSameDT=off  OutDataTypeStr=boolean
  Logical Operator8 : Logic  Operator=NOT  AllPortsSameDT=off  OutDataTypeStr=boolean
  Logical Operator9 : Logic  Operator=OR  AllPortsSameDT=off  OutDataTypeStr=boolean
  Switch : Switch  Criteria=u2 ~= 0  SaturateOnIntegerOverflow=off  InputSameDT=off
  Switch1 : Switch  Criteria=u2 ~= 0  SaturateOnIntegerOverflow=off  InputSameDT=off
  Unit Delay : UnitDelay  SampleTime=-1  HasFrameUpgradeWarning=on
  out : Outport
  wires:
  u/1 -> [u], Logical Operator/1
  R/1 -> [R], Logical Operator1/1
  IC/1 -> [IC], Logical Operator3/1, Logical Operator2/1
  Logical Operator3/1 -> Logical Operator1/2
  Logical Operator/1 -> Logical Operator4/1
  Logical Operator1/1 -> Logical Operator4/2
  [R] -> Logical Operator2/2
  Logical Operator2/1 -> [rst_true]
  dT_s/1 -> Divide/1, Add/1
  Constant/1 -> Divide/2
  Divide/1 -> [halfStep]
  DLY_s/1 -> Add1/1
  [halfStep] -> Add1/2
  Logical Operator4/1 -> Logical Operator8/1, Switch/2
  Constant1/1 -> Switch/1
  Add/1 -> Switch/3
  Switch/1 -> Unit Delay/1, GreaterThan/1
  Add1/1 -> GreaterThan/2
  Unit Delay/1 -> Add/2
  [u] -> Logical Operator5/1
  GreaterThan/1 -> Logical Operator6/1
  Logical Operator5/1 -> Logical Operator6/2
  Logical Operator6/1 -> Logical Operator7/2
  Logical Operator8/1 -> Logical Operator7/1
  DLYIC_Name/1 -> Logical Operator5/2
  [IC] -> DLYIC_Name/2
  Logical Operator7/1 -> Logical Operator9/2
  [rst_true] -> Logical Operator9/1
  Logical Operator9/1 -> Switch1/2
  Constant2/1 -> Switch1/1
  Constant3/1 -> Switch1/3
  Switch1/1 -> DLYIC_Name/1, out/1

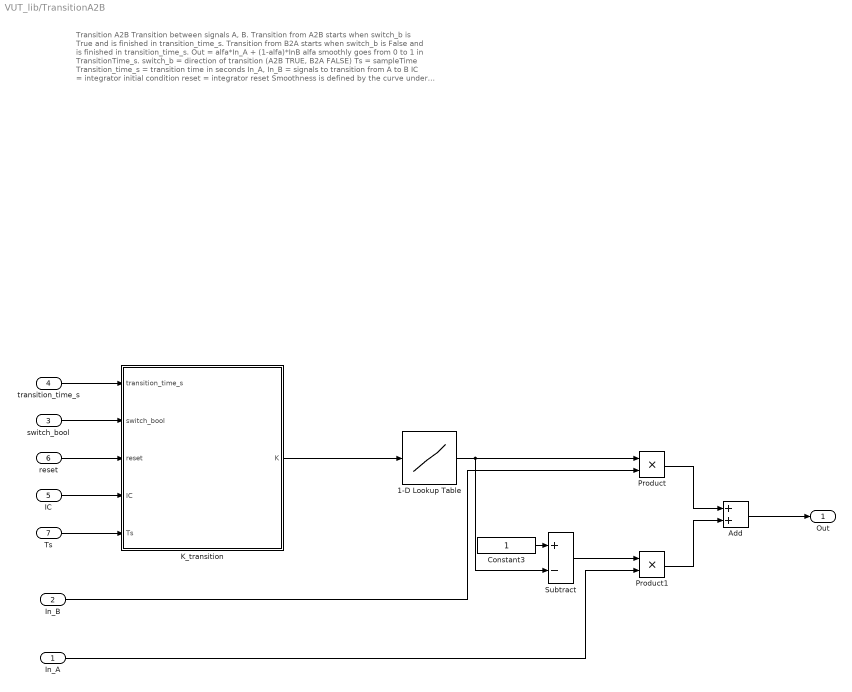
== system VUT_lib/TransitionA2B ==
  note: Transition A2B
      |
      | Transition between signals A, B.
      |
      | Transition from A2B starts when switch_b is True and
      | is finished in transition_time_s. Transition from B2A starts when
      | switch_b is False and is finished in transition_time_s.
      |
      | Out = alfa*In_A + (1-alfa)*InB
      |
      | alfa smoothly goes from 0 to 1 in TransitionTime_s.
      | switch_b = direction of transition (A2B TRUE, B2A FALSE)
      | Ts = sampleTime
      | Transition_time_s = transition time in seconds
      | In_A, In_B = signals to transition from A to B
      | IC = integrator initial condition
      | reset = integrator reset
      |
      | Smoothness is defined by the curve under the mask,
  In_A : Inport
  In_B : Inport  Port=2
  switch_bool : Inport  Port=3
  transition_time_s : Inport  Port=4
  IC : Inport  Port=5
  reset : Inport  Port=6
  Ts : Inport  Port=7
  1-D Lookup Table : Lookup_n-D  NumberOfTableDimensions=1  BreakpointsForDimension1=[0:0.01:1]  Table=[0,(tanh([-4.9:0.1:4.9])+1)/2,1]  InternalRulePriority=Speed  RndMeth=Simplest
  Add : Sum
  Constant3 : Constant  OutDataTypeStr=single
  K_transition : Subsystem
  Product : Product
  Product1 : Product
  Subtract : Sum  Inputs=+-
  Out : Outport
  wires:
  transition_time_s/1 -> K_transition/1(transition_time_s)
  switch_bool/1 -> K_transition/2(switch_bool)
  reset/1 -> K_transition/3(reset)
  IC/1 -> K_transition/4(IC)
  Ts/1 -> K_transition/5(Ts)
  K_transition/1(K) -> 1-D Lookup Table/1
  1-D Lookup Table/1 -> Product/1, Subtract/2
  Product/1 -> Add/1
  Product1/1 -> Add/2
  Add/1 -> Out/1
  In_B/1 -> Product/2
  In_A/1 -> Product1/2
  Subtract/1 -> Product1/1
  Constant3/1 -> Subtract/1

== system VUT_lib/deg_2_rad ==
  in : Inport
  Constant : Constant  Value=pi  OutDataTypeStr=Inherit: Inherit via back propagation
  Constant1 : Constant  Value=180
  Divide : Product  Inputs=*/  RndMeth=Zero  SaturateOnIntegerOverflow=on
  Product : Product
  out : Outport
  wires:
  Constant/1 -> Product/2
  in/1 -> Product/1
  Product/1 -> Divide/1
  Divide/1 -> out/1
  Constant1/1 -> Divide/2

== system VUT_lib/g_2_mps2 ==
  in : Inport
  Constant : Constant  Value=9.8066  OutDataTypeStr=Inherit: Inherit via back propagation
  Product : Product
  out : Outport
  wires:
  Constant/1 -> Product/2
  Product/1 -> out/1
  in/1 -> Product/1

== system VUT_lib/geometric_sum ==
  in1 : Inport
  in2 : Inport  Port=2
  Add : Sum
  Sqrt : Sqrt
  Square : Math  Operator=square
  Square1 : Math  Operator=square
  out : Outport
  wires:
  Square/1 -> Add/1
  in1/1 -> Square/1
  Square1/1 -> Add/2
  in2/1 -> Square1/1
  Sqrt/1 -> out/1
  Add/1 -> Sqrt/1

== system VUT_lib/kmph_2_mps ==
  in : Inport
  Constant : Constant  Value=3.6  OutDataTypeStr=Inherit: Inherit via back propagation
  Divide : Product  Inputs=*/  RndMeth=Zero  SaturateOnIntegerOverflow=on
  out : Outport
  wires:
  in/1 -> Divide/1
  Constant/1 -> Divide/2
  Divide/1 -> out/1

== system VUT_lib/m_2_mm ==
  in : Inport
  Constant : Constant  Value=1e3  OutDataTypeStr=Inherit: Inherit via back propagation
  Product : Product
  out : Outport
  wires:
  Constant/1 -> Product/2
  Product/1 -> out/1
  in/1 -> Product/1

== system VUT_lib/mm_2_m ==
  in : Inport
  Constant : Constant  Value=1e-3  OutDataTypeStr=Inherit: Inherit via back propagation
  Product : Product
  out : Outport
  wires:
  in/1 -> Product/1
  Constant/1 -> Product/2
  Product/1 -> out/1

== system VUT_lib/mps2_2_g ==
  in : Inport
  Constant : Constant  Value=0.101972  OutDataTypeStr=Inherit: Inherit via back propagation
  Product : Product
  out : Outport
  wires:
  Product/1 -> out/1
  in/1 -> Product/1
  Constant/1 -> Product/2

== system VUT_lib/mps_2_kmph ==
  in : Inport
  Constant : Constant  Value=3.6  OutDataTypeStr=Inherit: Inherit via back propagation
  Product : Product
  out : Outport
  wires:
  Constant/1 -> Product/2
  in/1 -> Product/1
  Product/1 -> out/1

== system VUT_lib/rad_2_deg ==
  in : Inport
  Constant : Constant  Value=180  OutDataTypeStr=Inherit: Inherit via back propagation
  Constant1 : Constant  Value=pi  OutDataTypeStr=single
  Divide : Product  Inputs=*/  RndMeth=Zero  SaturateOnIntegerOverflow=on
  Product : Product
  out : Outport
  wires:
  in/1 -> Product/1
  Constant/1 -> Product/2
  Product/1 -> Divide/1
  Constant1/1 -> Divide/2
  Divide/1 -> out/1

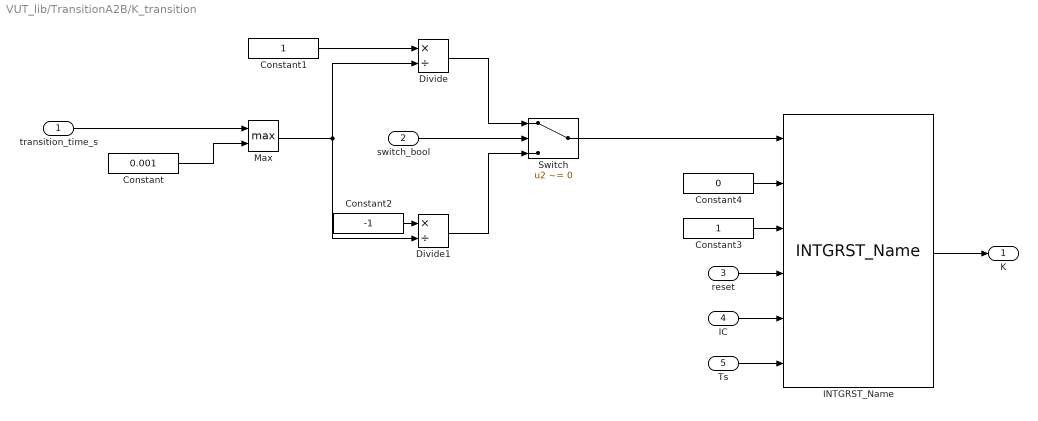
== system VUT_lib/TransitionA2B/K_transition ==
  transition_time_s : Inport
  switch_bool : Inport  Port=2
  reset : Inport  Port=3
  IC : Inport  Port=4
  Ts : Inport  Port=5
  Constant : Constant  Value=0.001  OutDataTypeStr=single
  Constant1 : Constant  OutDataTypeStr=single
  Constant2 : Constant  Value=-1  OutDataTypeStr=single
  Constant3 : Constant  OutDataTypeStr=single
  Constant4 : Constant  Value=0  OutDataTypeStr=single
  Divide : Product  Inputs=*/  RndMeth=Zero  SaturateOnIntegerOverflow=on
  Divide1 : Product  Inputs=*/  RndMeth=Zero  SaturateOnIntegerOverflow=on
  INTGRST_Name : $bdroot/INTGRST_Name  SystemSampleTime=-1  VariantActivationTime=update diagram  Latency=0  AutoFrameSizeCalculation=off
  Max : MinMax  Function=max  Inputs=2
  Switch : Switch  Criteria=u2 ~= 0  SaturateOnIntegerOverflow=off  InputSameDT=off
  K : Outport
  wires:
  switch_bool/1 -> Switch/2
  Constant/1 -> Max/2
  transition_time_s/1 -> Max/1
  Max/1 -> Divide/2, Divide1/2
  Constant1/1 -> Divide/1
  Constant2/1 -> Divide1/1
  Divide1/1 -> Switch/3
  Divide/1 -> Switch/1
  Switch/1 -> INTGRST_Name/1
  Constant4/1 -> INTGRST_Name/2
  Constant3/1 -> INTGRST_Name/3
  reset/1 -> INTGRST_Name/4
  IC/1 -> INTGRST_Name/5
  Ts/1 -> INTGRST_Name/6
  INTGRST_Name/1 -> K/1
